simulink model "week2_3"  (R2020b)
settings: Solver=VariableStepAuto  StartTime=0.0  StopTime=120  RelTol=1e-3
PreLoadFcn:
  | clear all;
  | close all;
  | clc;
  | m=1000;
  | b=50;
  | u=500;
settings Model: Creator=hp  LastModifiedBy=hp

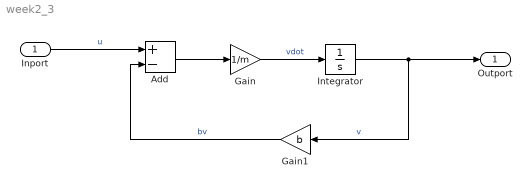
== system week2_3 ==
  Inport : Inport
  Add : Sum  Inputs=+-
  Gain : Gain  Gain=1/m
  Gain1 : Gain  Gain=b
  Integrator : Integrator
  Outport : Outport
  wires:
  Inport/1 -> Add/1  "u"
  Gain/1 -> Integrator/1  "vdot"
  Integrator/1 -> Outport/1, Gain1/1  "v"
  Add/1 -> Gain/1
  Gain1/1 -> Add/2  "bv"
